simulink model "ng_pv_dynamic_dbus_p_1_sm_ng"  (Simulink 8.8)
settings: Solver=ode4  StartTime=0.0  StopTime=inf  FixedStep=0.000125  RelTol=1e-3  EnableMultiTasking=on
PreLoadFcn:
  | Ts=125e-6;Core_Num = 0; np=1; nq=1; Vmin=.9;
PostLoadFcn:
  | Ts=125e-6;Core_Num = 0; np=1; nq=1; Vmin=.9;
InitFcn:
  | Ts=125e-6;Core_Num = 0; np=1; nq=1; Vmin=.9;
undefined symbols (not defined in the file or in its folder): another_event_name, DiscIntNeverNeededParam, I, j, Left, my_event_name, Right, type, V, X
libraries: powerlib x316, simulink_extras x78, powerlib_meascontrol x47, ssn_lib x9, opal_lib x5, powerlib_extras x3, simulink x3, artemis x1, rtio_opalrt_ml605ex1 x1, rtlab x1, rtio_spectracom x1
(part 11 of 11)

== matlab function SM_NG/Subsystem/Single-Phase Voltage Regulator1/Regulating logic ==
  data: tapNumberOut output double; vRelay input double; vRef input double; bandwidth input double; delayTime input double; clock input double; iTapNo parameter double
function tapNumberOut = Regulation_Logic(vRelay, vRef, bandwidth, delayTime, clock, iTapNo)

persistent timerStartTime; % Stores the start time of the timer.
if isempty(timerStartTime) 
timerStartTime = 0; 
end
persistent isTimerOn; % A flag to show that the timer is on. 1 means the timer is on.
if isempty(isTimerOn) 
isTimerOn = 0; 
end
persistent tapNumber; % Stores the tap number
if isempty(tapNumber) 
tapNumber = iTapNo; 
end

% Start the timer if the voltage is out of range.
if abs(vRelay - vRef) > (bandwidth / 2) && (isTimerOn == 0)
    timerStartTime = clock; 
    isTimerOn = 1;
end

% If the voltage is back to normal before the delay time is passed, stop the timer.
if (clock <= (timerStartTime + delayTime)) && (isTimerOn == 1) && (abs(vRelay - vRef) <= (bandwidth / 2))
    isTimerOn = 0;
end

% If the timer has passed the delay and the voltage is still out of range, change the tap number and reset the timer.
if (clock >= (timerStartTime + delayTime)) && (isTimerOn == 1) && (abs(vRelay - vRef) > (bandwidth / 2))
    if vRelay > vRef
        tapNumber = tapNumber - 1;
        if tapNumber < -16,  tapNumber = -16; end
        isTimerOn = 0;      
    else
        tapNumber = tapNumber + 1;
        if tapNumber > 16,  tapNumber = 16; end
        isTimerOn = 0;        
    end
end

tapNumberOut = tapNumber;

== matlab function SM_NG/Subsystem/Single-Phase Voltage Regulator2/Regulating logic ==
  data: tapNumberOut output double; vRelay input double; vRef input double; bandwidth input double; delayTime input double; clock input double; iTapNo parameter double
function tapNumberOut = Regulation_Logic(vRelay, vRef, bandwidth, delayTime, clock, iTapNo)

persistent timerStartTime; % Stores the start time of the timer.
if isempty(timerStartTime) 
timerStartTime = 0; 
end
persistent isTimerOn; % A flag to show that the timer is on. 1 means the timer is on.
if isempty(isTimerOn) 
isTimerOn = 0; 
end
persistent tapNumber; % Stores the tap number
if isempty(tapNumber) 
tapNumber = iTapNo; 
end

% Start the timer if the voltage is out of range.
if abs(vRelay - vRef) > (bandwidth / 2) && (isTimerOn == 0)
    timerStartTime = clock; 
    isTimerOn = 1;
end

% If the voltage is back to normal before the delay time is passed, stop the timer.
if (clock <= (timerStartTime + delayTime)) && (isTimerOn == 1) && (abs(vRelay - vRef) <= (bandwidth / 2))
    isTimerOn = 0;
end

% If the timer has passed the delay and the voltage is still out of range, change the tap number and reset the timer.
if (clock >= (timerStartTime + delayTime)) && (isTimerOn == 1) && (abs(vRelay - vRef) > (bandwidth / 2))
    if vRelay > vRef
        tapNumber = tapNumber - 1;
        if tapNumber < -16,  tapNumber = -16; end
        isTimerOn = 0;      
    else
        tapNumber = tapNumber + 1;
        if tapNumber > 16,  tapNumber = 16; end
        isTimerOn = 0;        
    end
end

tapNumberOut = tapNumber;

== matlab function SM_NG/Subsystem/Single-Phase Voltage Regulator3/Regulating logic ==
  data: tapNumberOut output double; vRelay input double; vRef input double; bandwidth input double; delayTime input double; clock input double; iTapNo parameter double
function tapNumberOut = Regulation_Logic(vRelay, vRef, bandwidth, delayTime, clock, iTapNo)

persistent timerStartTime; % Stores the start time of the timer.
if isempty(timerStartTime) 
timerStartTime = 0; 
end
persistent isTimerOn; % A flag to show that the timer is on. 1 means the timer is on.
if isempty(isTimerOn) 
isTimerOn = 0; 
end
persistent tapNumber; % Stores the tap number
if isempty(tapNumber) 
tapNumber = iTapNo; 
end

% Start the timer if the voltage is out of range.
if abs(vRelay - vRef) > (bandwidth / 2) && (isTimerOn == 0)
    timerStartTime = clock; 
    isTimerOn = 1;
end

% If the voltage is back to normal before the delay time is passed, stop the timer.
if (clock <= (timerStartTime + delayTime)) && (isTimerOn == 1) && (abs(vRelay - vRef) <= (bandwidth / 2))
    isTimerOn = 0;
end

% If the timer has passed the delay and the voltage is still out of range, change the tap number and reset the timer.
if (clock >= (timerStartTime + delayTime)) && (isTimerOn == 1) && (abs(vRelay - vRef) > (bandwidth / 2))
    if vRelay > vRef
        tapNumber = tapNumber - 1;
        if tapNumber < -16,  tapNumber = -16; end
        isTimerOn = 0;      
    else
        tapNumber = tapNumber + 1;
        if tapNumber > 16,  tapNumber = 16; end
        isTimerOn = 0;        
    end
end

tapNumberOut = tapNumber;
